simulink model "single_dmp_test"  (R2020b)
settings: Solver=ode8  StartTime=0.0  StopTime=10.0  FixedStep=0.005  RelTol=1e-3
undefined symbols (not defined in the file): cc_new, D, K, left_0, tau1, weight, width_new
settings Model: Creator=10788  LastModifiedBy=10788
settings OptimizationCC: DefaultParameterBehavior=Inlined  UseDivisionForNetSlopeComputation=on  GainParamInheritBuiltInType=on  UseFloatMulNetSlope=on  InlineInvariantSignals=on  PassReuseOutputArgsAs=Individual arguments  ZeroExternalMemoryAtStartup=off  ZeroInternalMemoryAtStartup=off  NoFixptDivByZeroProtection=on  EfficientFloat2IntCast=on  LifeSpan=1  OptimizeBlockOrder=speed  DifferentSizesBufferReuse=on  EfficientTunableParamExpr=on
settings DebuggingCC: ParameterTunabilityLossMsg=error
settings HardwareCC: ProdLongLongMode=on
settings SFSimCC: MATLABDynamicMemAlloc=off  SimTargetLang=C++
settings RTWCC: Description=Embedded Coder  SystemTargetFile=ert.tlc  TemplateMakefile=ert_default_tmf  GenerateReport=on  LaunchReport=on  TargetLang=C++
settings CodeAppCC: ForceParamTrailComments=on  IgnoreCustomStorageClasses=off  OperatorAnnotations=on  SimulinkDataObjDesc=on  SFDataObjDesc=on  CustomSymbolStrGlobalVar=rt$N$M  CustomSymbolStrType=$N$M  CustomSymbolStrFcn=$N$M$F  CustomSymbolStrMacro=$N$M  InsertBlockDesc=on
settings ERTTargetCC: TargetLangStandard=C++03 (ISO)  GenerateSampleERTMain=on  IncludeMdlTerminateFcn=off  CombineSignalStateStructs=on  SupportAbsoluteTime=off  CodeInterfacePackaging=C++ class  SupportComplex=off  SupportContinuousTime=on  SupportNonInlinedSFcns=on  InlinedParameterPlacement=NonHierarchical  RootIOFormat=Structure reference  ERTCustomFileTemplate=example_file_process.tlc  ERTFilePackagingFormat=CompactWithDataFile

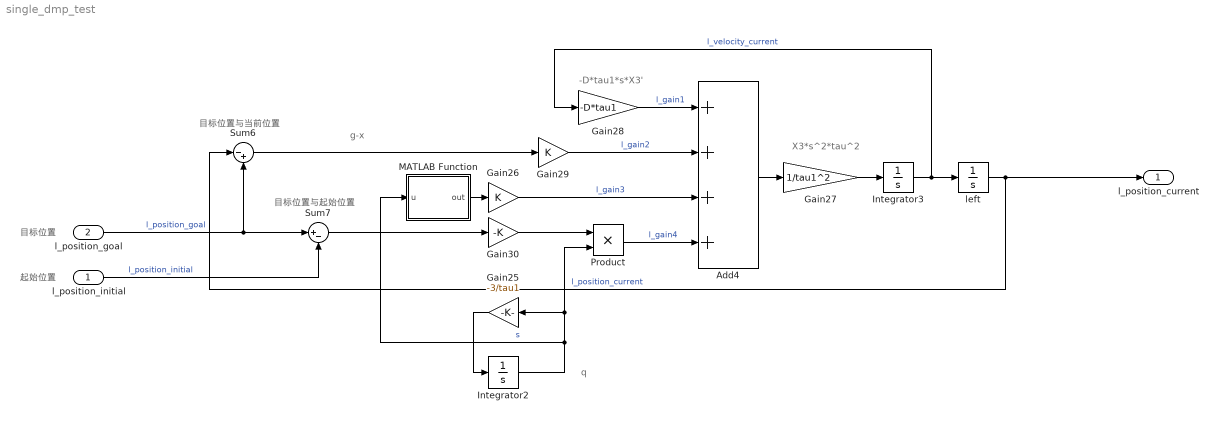
== system single_dmp_test ==
  note: 目标位置与当前位置
  note: 起始位置
  note: X3*s^2*tau^2
  note: 目标位置
  note: 目标位置与起始位置
  note: -D*tau1*s*X3'
  note: g-x
  note: q
  l_position_initial : Inport  OutDataTypeStr=double  PortDimensions=3
  l_position_goal : Inport  Port=2  OutDataTypeStr=double  PortDimensions=3
  Add4 : Sum  Inputs=++++
  Gain25 : Gain  Gain=-3/tau1
  Gain26 : Gain  Gain=K
  Gain27 : Gain  Gain=1/tau1^2
  Gain28 : Gain  Gain=-D*tau1
  Gain29 : Gain  Gain=K
  Gain30 : Gain  Gain=-K
  Integrator2 : Integrator  InitialCondition=1
  Integrator3 : Integrator
  MATLAB Function : MATLAB Function  TreatAsAtomicUnit=on
  Product : Product
  Sum6 : Sum  Inputs=|-+
  Sum7 : Sum  Inputs=|+-
  left : Integrator  InitialCondition=left_0
  l_position_current : Outport
  wires:
  Add4/1 -> Gain27/1
  Product/1 -> Add4/4  "l_gain4"
  Gain25/1 -> Integrator2/1
  Integrator3/1 -> Gain28/1, left/1  "l_velocity_current"
  Gain27/1 -> Integrator3/1
  Sum7/1 -> Gain30/1
  Gain30/1 -> Product/1
  Integrator2/1 -> Product/2, Gain25/1, MATLAB Function/1(u)  "s"
  MATLAB Function/1(out) -> Gain26/1
  Sum6/1 -> Gain29/1
  l_position_goal/1 -> Sum7/1, Sum6/2  "l_position_goal"
  Gain29/1 -> Add4/2  "l_gain2"
  left/1 -> l_position_current/1, Sum6/1  "l_position_current"
  l_position_initial/1 -> Sum7/2  "l_position_initial"
  Gain26/1 -> Add4/3  "l_gain3"
  Gain28/1 -> Add4/1  "l_gain1"

== matlab function single_dmp_test/MATLAB Function ==
  data: u input; out output; width_new parameter; weight parameter; cc_new parameter
function out = fcn(u, width_new, weight, cc_new)


% if(u>2.5)
%     y=1;
% elseif(u>=0&&u<=2.5)
%     y=0;
% else
%         y=-1;
% end


tem=exp(-width_new.*(u-cc_new).^2)';
y=(weight * tem * u) / sum(tem) ;

out = y;
